simulink model "Modelo_Sistema_Realimentado_PI_Rampa"  (R2018b)
settings: Solver=FixedStepAuto  StartTime=0.0  StopTime=20.0  FixedStep=0.01  RelTol=0.001
libraries: simulink x1
settings Model: Creator=rafab  LastModifiedBy=rafab

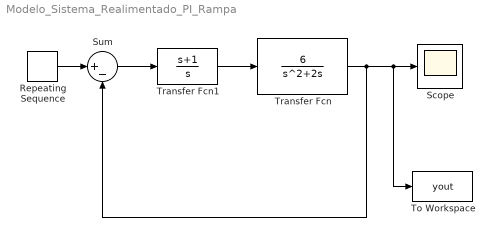
== system Modelo_Sistema_Realimentado_PI_Rampa ==
  Repeating Sequence : simulink/Sources/Repeating Sequence  rep_seq_t=[0 2]  rep_seq_y=[0 20]
  Scope : Scope
  Sum : Sum  Inputs=|+-
  To Workspace : ToWorkspace  VariableName=yout  SampleTime=-1
      settings: Save2DSignal=2-D array (concatenate along first dimension)
  Transfer Fcn : TransferFcn  Numerator=[6]  Denominator=[1 2 0]
  Transfer Fcn1 : TransferFcn  Numerator=[1 1]  Denominator=[0 1 0]
  wires:
  Transfer Fcn/1 -> To Workspace/1, Scope/1, Sum/2
  Repeating Sequence/1 -> Sum/1
  Sum/1 -> Transfer Fcn1/1
  Transfer Fcn1/1 -> Transfer Fcn/1
